simulink model "rtwdemo_international"  (Simulink 7.4)
settings: Solver=FixedStepDiscrete  StartTime=0.0  StopTime=48  FixedStep=1  RelTol=1e-3
PreLoadFcn:
  | rtwdemo_international_data
values from neighbouring files (symbols this model uses):
  LIMIT = Simulink.Parameter    [rtwdemo_international_data.m]
libraries: rtwdemowidgets x1
Description:
  | 日本語で記述したモデルの説明
settings Model: Creator=The MathWorks Inc.  ModifiedHistory=日本語で記述したモデルの履歴  ParamWorkspaceSource=ReferencedWorkspace  CovMetricSettings=d  ExtModeTrigMode=oneshot  ExtModeArmWhenConnect=off  ExtModeAutoUpdateStatusClock=off
settings DataIOCC: LimitDataPoints=off  SaveFormat=StructureWithTime  SaveOutput=off  SaveTime=off  SignalLoggingName=sigsOut
settings OptimizationCC: InlineParams=on  InlineInvariantSignals=on  StateBitsets=on  DataBitsets=on  UseTempVars=on  ZeroExternalMemoryAtStartup=off  ZeroInternalMemoryAtStartup=off  NoFixptDivByZeroProtection=on  EfficientFloat2IntCast=on  OptimizeModelRefInitCode=on  LifeSpan=1  BufferReusableBoundary=off
settings DebuggingCC: SaveWithParameterizedLinksMsg=none  CheckExecutionContextPreStartOutputMsg=on  CheckExecutionContextRuntimeOutputMsg=on  SignalResolutionControl=TryResolveAllWithWarning  SolverPrmCheckMsg=none  MultiTaskDSMMsg=warning  MultiTaskCondExecSysMsg=none  IntegerOverflowMsg=none  StrictBusMsg=None
settings HardwareCC: ProdIntDivRoundTo=Zero  ProdEndianess=LittleEndian  ProdHWDeviceType=Specified  TargetHWDeviceType=32-bit Generic
settings ModelReferenceCC: UpdateModelReferenceTargets=IfOutOfDate
settings SFSimCC: SimGenerateEmlReport=off
settings RTWCC: SystemTargetFile=ert.tlc  TLCOptions=-p0 -aWarnNonSaturatedBlocks=0  TemplateMakefile=ert_default_tmf  Description=Real-Time Workshop Embedded Coder  GenerateReport=on  RTWVerbose=off  ProcessScript=ert_make_rtw_hook  IncludeHyperlinkInReport=on  LaunchReport=on  GenerateTraceInfo=on  GenerateTraceReport=on  GenerateTraceReportSl=on  GenerateTraceReportSf=on  GenerateTraceReportEml=on
settings CodeAppCC: ForceParamTrailComments=on  IgnoreCustomStorageClasses=off  SimulinkDataObjDesc=on  SFDataObjDesc=on  CustomSymbolStrGlobalVar=rt$N$M  CustomSymbolStrType=$N$M  CustomSymbolStrFcn=$N$M$F  CustomSymbolStrMacro=$N$M  InsertBlockDesc=on
settings ERTTargetCC: MultiwordLength=2048  GenerateSampleERTMain=on  IncludeMdlTerminateFcn=off  SupportNonFinite=off  SupportComplex=off  InlinedParameterPlacement=NonHierarchical  ERTSrcFileBannerTemplate=rtwdemo_international.cgt  ERTHdrFileBannerTemplate=rtwdemo_international.cgt  ERTDataSrcFileTemplate=rtwdemo_international.cgt  ERTDataHdrFileTemplate=rtwdemo_international.cgt  ERTCustomFileTemplate=rtwdemofileprocess_international.tlc  ConvertIfToSwitch=off

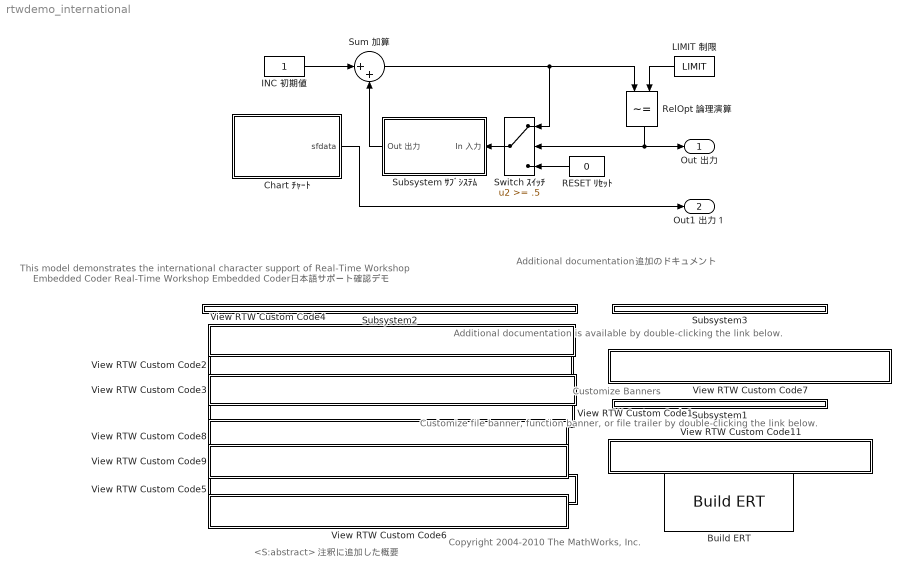
== system rtwdemo_international ==
  note: This model demonstrates the international character
      | support of Real-Time Workshop Embedded Coder
      | Real-Time Workshop Embedded Coder
      | 日本語サポート確認デモ
  note: Additional documentation
      | 追加のドキュメント
  note: Additional documentation is available
      | by double-clicking the link below.
  note: Customize Banners
  note: Customize file banner, function banner,
      | or file trailer by double-clicking the link below.
  note: <S:abstract> 注釈に追加した概要
  note: Copyright 2004-2010 The MathWorks, Inc.
  Build ERT : rtwdemowidgets/Build ERT  SystemSampleTime=-1  attrib_overrides={'ERTCustomFileTemplate','ERTSrcFileBannerTemplate','ERTHdrFileBannerTemplate','ERTDataSrcFileTemplate','ERTDataHdrFileTemplate'}
  Chart ﾁｬｰﾄ : Stateflow chart
  INC 初期値 : Constant  OutDataTypeMode=uint8  OutDataType=sfix(16)  OutScaling=2^0  OutDataTypeStr=uint8
  LIMIT 制限 : Constant  Value=LIMIT  OutDataTypeMode=uint8  OutDataType=sfix(16)  OutScaling=2^0  OutDataTypeStr=uint8
  "RESET ﾘｾｯﾄ " : Constant  Value=0  OutDataTypeMode=uint8  OutDataType=sfix(16)  OutScaling=2^0  OutDataTypeStr=uint8
  RelOpt 論理演算 : RelationalOperator  Operator=~=  InputSameDT=on
  Subsystem ｻﾌﾞｼｽﾃﾑ : Subsystem  TreatAsAtomicUnit=on
  Subsystem1 : Subsystem
  Subsystem2 : Subsystem
  Subsystem3 : Subsystem
  Sum 加算 : Sum  Inputs=|++  OutDataType=sfix(16)  OutScaling=2^0  InputSameDT=on  OutDataTypeStr=Inherit: Same as first input
  Switch ｽｲｯﾁ : Switch  Description=|  Threshold=.5  SaturateOnIntegerOverflow=on  InputSameDT=on
      | Japanese comments in block description:
      | ﾌﾞﾛｯｸの概要に記述された日本語ｺﾒﾝﾄ
  View RTW Custom Code1 : Subsystem
      mask init:
      | pos    = get_param(gcb, 'Position');
      | width  = pos(3) - pos(1);
      | height = pos(4) - pos(2);
      | 
      | 
      | % Compute arrow coordinates
      | arrowW = width  / 20;
      | arrowH = height / 2.5;
      | arrowX = width  / 50;
      | arrowY = height / 3;
      | arrowXvec = [arrowX, arrowX, arrowX + arrowW];
      | arrowYvec = [arrowY, arrowY + arrowH, arrowY + arrowH / 2];
      | 
      | % Compute text position
      | textXbuff = width / 30;
      | textX  = arrowX + arrowW + textXbuff;
      | textY  = height / 2;
      settings: OpenFcn=|
      | rt=sfroot;
      | sfTransObj = rt.find('-isa','Stateflow.Transition', '-and', 'Path',[bdroot '/Chart ﾁｬｰﾄ']);
      | sfTransObj(1).dialog;   clear rt sfTransObj;
      mask Display:
      | patch(arrowXvec, arrowYvec);
      | text(textX, textY, 'Stateflow Object Description      ');
  View RTW Custom Code11 : Subsystem
      mask init: same as rtwdemo_international/View RTW Custom Code1
      settings: OpenFcn=edit rtwdemo_international.cgt
      mask Display:
      | patch(arrowXvec, arrowYvec);
      | text(textX, textY, 'Customize banners via code templates');
  View RTW Custom Code2 : Subsystem
      mask init: same as rtwdemo_international/View RTW Custom Code1
      settings: OpenFcn=|
      | block=[bdroot, '/Switch ｽｲｯﾁ'];
      | hilite_system(block);
      | open_system(block, 'property'); clear block;
      mask Display:
      | patch(arrowXvec, arrowYvec);
      | text(textX, textY, 'Simulink Block Description');
  View RTW Custom Code3 : Subsystem
      mask init: same as rtwdemo_international/View RTW Custom Code1
      settings: OpenFcn=|
      | block=[bdroot, '/Chart ﾁｬｰﾄ'];
      | open_system(block);    clear block;
      mask Display:
      | patch(arrowXvec, arrowYvec);
      | text(textX, textY, 'Stateflow Custom Comments');
  View RTW Custom Code4 : Subsystem
      mask init: same as rtwdemo_international/View RTW Custom Code1
      settings: OpenFcn=|
      | block=[bdroot, '/Switch ｽｲｯﾁ'];
      | hilite_system(block);     clear block;
      mask Display:
      | patch(arrowXvec, arrowYvec);
      | text(textX, textY, 'Simulink Block Name');
  View RTW Custom Code5 : Subsystem
      mask init: same as rtwdemo_international/View RTW Custom Code1
      settings: OpenFcn=|
      | slCfgPrmDlg(bdroot,'Open');
      | slCfgPrmDlg(bdroot,'TurnToPage','Templates');
      mask Display:
      | patch(arrowXvec, arrowYvec);
      | text(textX, textY, 'RTW-EC Code Template File');
  View RTW Custom Code6 : Subsystem
      mask init: same as rtwdemo_international/View RTW Custom Code1
      settings: OpenFcn=|
      | slCfgPrmDlg(bdroot,'Open');
      | slCfgPrmDlg(bdroot,'TurnToPage','Templates');
      mask Display:
      | patch(arrowXvec, arrowYvec);
      | text(textX, textY, 'Custom TLC File ');
  View RTW Custom Code7 : Subsystem
      mask init: same as rtwdemo_international/View RTW Custom Code1
      settings: OpenFcn=helpview([docroot '/toolbox/rtw/helptargets.map'], 'rtw_non_us_ascii_support')
      mask Display:
      | patch(arrowXvec, arrowYvec);
      | text(textX, textY, 'RTW international support documentation');
  View RTW Custom Code8 : Subsystem
      mask init: same as rtwdemo_international/View RTW Custom Code1
      settings: OpenFcn=DAStudio.Dialog(LIMIT);
      mask Display:
      | patch(arrowXvec, arrowYvec);
      | text(textX, textY, 'Simulink Parameter Object Description');
  View RTW Custom Code9 : Subsystem
      mask init: same as rtwdemo_international/View RTW Custom Code1
      settings: OpenFcn=DAStudio.Dialog(mpts1);
      mask Display:
      | patch(arrowXvec, arrowYvec);
      | text(textX, textY, 'MPT Signal Object Description');
  Out 出力 : Outport  OutDataType=sfix(16)  OutScaling=2^0
  Out1 出力１ : Outport  Port=2  OutDataType=sfix(16)  OutScaling=2^0
  wires:
  INC 初期値/1 -> Sum 加算/1
  Subsystem ｻﾌﾞｼｽﾃﾑ/1(Out 出力) -> Sum 加算/2
  Switch ｽｲｯﾁ/1 -> Subsystem ｻﾌﾞｼｽﾃﾑ/1(In 入力)
  Sum 加算/1 -> Switch ｽｲｯﾁ/1, RelOpt 論理演算/1
  LIMIT 制限/1 -> RelOpt 論理演算/2
  "RESET ﾘｾｯﾄ "/1 -> Switch ｽｲｯﾁ/3
  RelOpt 論理演算/1 -> Switch ｽｲｯﾁ/2, Out 出力/1
  Chart ﾁｬｰﾄ/1(sfdata) -> Out1 出力１/1

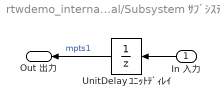
== system rtwdemo_international/Subsystem ｻﾌﾞｼｽﾃﾑ ==
  In 入力 : Inport  OutDataType=sfix(16)  OutScaling=2^0
  UnitDelay ﾕﾆｯﾄﾃﾞｨﾚｲ : UnitDelay  StateIdentifier=X
  Out 出力 : Outport  OutDataType=sfix(16)  OutScaling=2^0
  wires:
  In 入力/1 -> UnitDelay ﾕﾆｯﾄﾃﾞｨﾚｲ/1
  UnitDelay ﾕﾆｯﾄﾃﾞｨﾚｲ/1 -> Out 出力/1  "mpts1"

== system rtwdemo_international/Subsystem1 ==

== system rtwdemo_international/Subsystem2 ==

== system rtwdemo_international/Subsystem3 ==

== system rtwdemo_international/View RTW Custom Code1 ==

== system rtwdemo_international/View RTW Custom Code11 ==

== system rtwdemo_international/View RTW Custom Code2 ==

== system rtwdemo_international/View RTW Custom Code3 ==

== system rtwdemo_international/View RTW Custom Code4 ==

== system rtwdemo_international/View RTW Custom Code5 ==

== system rtwdemo_international/View RTW Custom Code6 ==

== system rtwdemo_international/View RTW Custom Code7 ==

== system rtwdemo_international/View RTW Custom Code8 ==

== system rtwdemo_international/View RTW Custom Code9 ==

== stateflow chart Chart ﾁｬｰﾄ ==
  state State
    entry: a = a +2 ; /* Japanese comments in State example 1 */
    du: a++;            /*ステートに記述した日本語コメント例 １ */
    /*
    Japanese comments in State example 2
    ステートに記述した日本語コメント例２
    ﾊﾝｶｸｶﾀｶﾅ
    Ｗｉｄｅ Ｓｐａｃｅｄ Ｅｎｇｌｉｓｈ
    ひらがな
    カタカナ
    漢字
    */
    State -> State [order 1] : [a/2==0]
  note: <S:Description> Stateflow日本語サポート確認
  (default) -> State : { a = 1; /* Japanese comments in Transition example 1
      |                 ﾄﾗﾝｼﾞｼｮﾝに記述した日本語コメント例１     */}
    settings: description=|
        | Stateflow object descriptions:
        | Stateflow オブジェクトの概要に記述された日本語ｺﾒﾝﾄ
  State -> State [order 1] : [a/6 == 0]{a=0;} /* Japanese comments in Transition example 2
      |                          ﾄﾗﾝｼﾞｼｮﾝに記述した日本語コメント例２      */
    settings: description=日本
  data: sfdata output double; a local int32
  data sfdata settings: description=Stateflow data object descriptions: Stateflow データオブジェクト説明
